simulink model "Longitudinal_new_modified"  (R2025b)
settings: Solver=VariableStepAuto  StartTime=0.0  StopTime=4  MaxStep=0.001  RelTol=1e-3
undefined symbols (not defined in the file): car, rad, s, Tau_1, Tau_2, Tau_3, Tau_4, Tau_EM, tyre
libraries: aerolibconvert2 x3, simulink x2
(part 2 of 2)

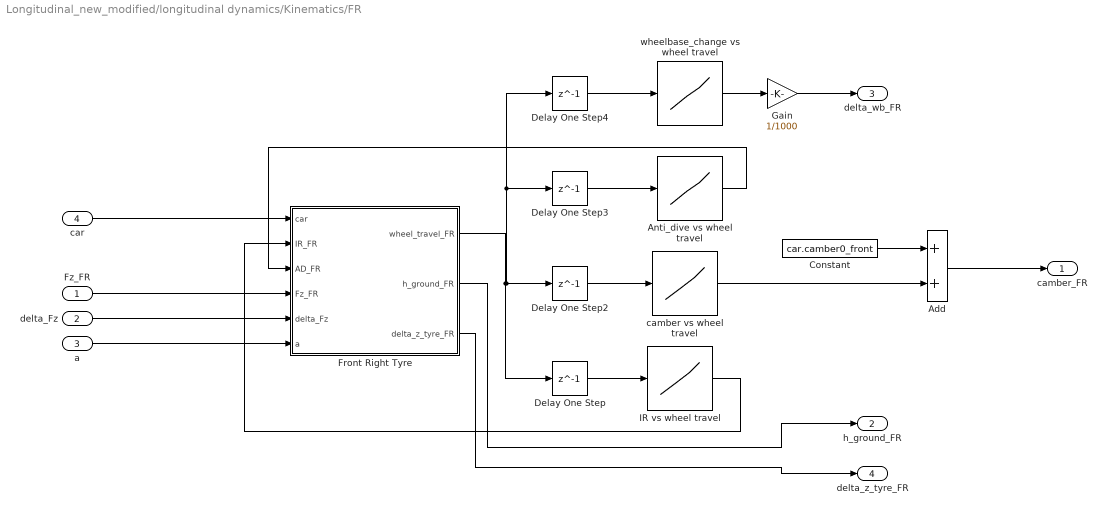
== system Longitudinal_new_modified/longitudinal dynamics/Kinematics/FR ==
  Fz_FR : Inport
  delta_Fz : Inport  Port=2
  a : Inport  Port=3
  car : Inport  Port=4
  Add : Sum
  Anti_dive vs wheel travel : Lookup_n-D  NumberOfTableDimensions=1  BreakpointsForDimension1=[-20;-19;-18;-17;-16;-15;-14;-13;-12;-11;-10;-9;-8;-7;-6;-5;-4;-3;-2;-1;0;1;2;3;4;5;6;7;8;9;10;11;12;13;14;15;16;17;18;19;20;21;22;23;24;25;26;27;28;29;30;31;32;33;34;35;36;37;38;39;40;41;42;43;44;45;46;47;48;49;50;51;52;53;54;55;56;57;58;59;60;61;62;63;64;65;66;67;68;69;70;71;72;73;74;75]  Table=[56.11;56.3;56.5;56.69;56.89;57.08;57.28;57.48;57.68;57.88;58.09;58.29;58.5;58.7;58.91;59.12;59.33;59.54;59.76;59.97;60.19;60.4;60.62;60.84;61.06;61.29;61.51;61.74;61.96;62.19;62.42;62.65;62.88;63.12;63.35;63.59;63.83;64.06999999999999;64.31;64.56;64.8;65.05;65.3;65.55;65.8;66.05;66.31;66.56999999999999;66.83;67.09;67.34999999999999;67.61;67.88;68.15000000000001;68.42;68.69;68.95999999999999;69.23999999999999;69.52;69.8;70.08;70.36;70.65000000000001;70.94;71.23;71.52;71.81;72.11;72.41;72.70999999999999;73.02;73.31999999999999;73.63;73.94;74.25;74.56999999999999;74.89;75.20999999999999;75.53;75.84999999999999;76.18000000000001;76.51000000000001;76.84999999999999;77.18000000000001;77.52;77.86;78.20999999999999;78.55;78.90000000000001;79.26000000000001;79.61;79.97;80.33;80.7;81.06;81.43000000000001]  InternalRulePriority=Speed  RndMeth=Simplest
  Constant : Constant  Value=car.camber0_front
  Delay One Step{,2..4} (4 alike) : Delay  DelayLength=1
  Front Right Tyre : MATLAB Function  TreatAsAtomicUnit=on
  Gain : Gain  Gain=1/1000
  IR vs wheel travel : Lookup_n-D  NumberOfTableDimensions=1  BreakpointsForDimension1=[-20;-19;-18;-17;-16;-15;-14;-13;-12;-11;-10;-9;-8;-7;-6;-5;-4;-3;-2;-1;0;1;2;3;4;5;6;7;8;9;10;11;12;13;14;15;16;17;18;19;20;21;22;23;24;25;26;27;28;29;30;31;32;33;34;35;36;37;38;39;40;41;42;43;44;45;46;47;48;49;50;51;52;53;54;55;56;57;58;59;60;61;62;63;64;65;66;67;68;69;70;71;72;73;74;75]  Table=[0.5620000000000001;0.562105263157895;0.562222222222222;0.5623529411764711;0.5625;0.562666666666667;0.5628571428571429;0.563076923076923;0.563333333333333;0.562727272727273;0.5629999999999999;0.563333333333333;0.5625;0.5628571428571429;0.563333333333333;0.5639999999999999;0.5625;0.563333333333333;0.5649999999999999;0.5600000000000001;0.5600000000000001;0.5600000000000001;0.5649999999999999;0.563333333333333;0.5625;0.5620000000000001;0.561666666666667;0.5614285714285711;0.56125;0.561111111111111;0.5610000000000001;0.560909090909091;0.560833333333333;0.560769230769231;0.5607142857142861;0.560666666666667;0.5600000000000001;0.5600000000000001;0.559444444444444;0.559473684210526;0.5590000000000001;0.559047619047619;0.558636363636364;0.558260869565217;0.5579166666666669;0.5576;0.5573076923076919;0.557037037037037;0.556785714285714;0.556551724137931;0.556333333333333;0.555806451612903;0.555625;0.555151515151515;0.554705882352941;0.554571428571429;0.554166666666667;0.553783783783784;0.553421052631579;0.553076923076923;0.55275;0.5524390243902439;0.551904761904762;0.551627906976744;0.551136363636364;0.550888888888889;0.550434782608696;0.55;0.549583333333333;0.549183673469388;0.5488;0.54843137254902;0.548076923076923;0.547547169811321;0.5472222222222221;0.546727272727273;0.546428571428571;0.545964912280702;0.54551724137931;0.545084745762712;0.544666666666667;0.544262295081967;0.543870967741935;0.543492063492063;0.543125;0.5426153846153851;0.542272727272727;0.5417910447761189;0.541323529411765;0.587971014492754;0.585285714285714;0.582676056338028;0.580277777777778;0.577808219178082;0.575405405405405;0.5732]  InternalRulePriority=Speed  RndMeth=Simplest
  camber vs wheel travel : Lookup_n-D  NumberOfTableDimensions=1  BreakpointsForDimension1=[-20;-19;-18;-17;-16;-15;-14;-13;-12;-11;-10;-9;-8;-7;-6;-5;-4;-3;-2;-1;0;1;2;3;4;5;6;7;8;9;10;11;12;13;14;15;16;17;18;19;20;21;22;23;24;25;26;27;28;29;30;31;32;33;34;35;36;37;38;39;40;41;42;43;44;45;46;47;48;49;50;51;52;53;54;55;56;57;58;59;60;61;62;63;64;65;66;67;68;69;70;71;72;73;74;75]  Table=[0.94910000000000005;0.90229999999999999;0.85550000000000004;0.80859999999999999;0.76160000000000005;0.71450000000000002;0.66739999999999999;0.62019999999999997;0.57299999999999995;0.52569999999999995;0.4783;0.43080000000000002;0.38319999999999999;0.33560000000000001;0.28789999999999999;0.24010000000000001;0.1923;0.14430000000000001;0.096299999999999997;0.0482;0;-0.048300000000000003;-0.096600000000000005;-0.14510000000000001;-0.19359999999999999;-0.2422;-0.29089999999999999;-0.3397;-0.3886;-0.43759999999999999;-0.48670000000000002;-0.53580000000000005;-0.58509999999999995;-0.63439999999999996;-0.68389999999999995;-0.73340000000000005;-0.78310000000000002;-0.83279999999999998;-0.88270000000000004;-0.93259999999999998;-0.98270000000000002;-1.0327999999999999;-1.0831;-1.1334;-1.1839;-1.2344999999999999;-1.2851999999999999;-1.3360000000000001;-1.3869;-1.4379;-1.4890000000000001;-1.5403;-1.5915999999999999;-1.6431;-1.6947000000000001;-1.7464;-1.7982;-1.8501000000000001;-1.9021999999999999;-1.9543999999999999;-2.0066999999999999;-2.0590999999999999;-2.1116999999999999;-2.1644000000000001;-2.2172000000000001;-2.2700999999999998;-2.3231999999999999;-2.3763999999999998;-2.4297;-2.4830999999999999;-2.5367000000000002;-2.5903999999999998;-2.6442999999999999;-2.6983000000000001;-2.7524000000000002;-2.8067000000000002;-2.8611;-2.9156;-2.9702999999999999;-3.0251000000000001;-3.0800999999999998;-3.1352000000000002;-3.1903999999999999;-3.2458;-3.3014000000000001;-3.3571;-3.4129;-3.4689000000000001;-3.5251000000000001;-3.5813999999999999;-3.6377999999999999;-3.6945000000000001;-3.7511999999999999;-3.8081;-3.8652000000000002;-3.9224999999999999]  InternalRulePriority=Speed  RndMeth=Simplest
  wheelbase_change vs wheel travel : Lookup_n-D  NumberOfTableDimensions=1  BreakpointsForDimension1=[-20;-19;-18;-17;-16;-15;-14;-13;-12;-11;-10;-9;-8;-7;-6;-5;-4;-3;-2;-1;0;1;2;3;4;5;6;7;8;9;10;11;12;13;14;15;16;17;18;19;20;21;22;23;24;25;26;27;28;29;30;31;32;33;34;35;36;37;38;39;40;41;42;43;44;45;46;47;48;49;50;51;52;53;54;55;56;57;58;59;60;61;62;63;64;65;66;67;68;69;70;71;72;73;74;75]  Table=[0.25;0.23999999999999999;0.22;0.20999999999999999;0.19;0.17999999999999999;0.16;0.14999999999999999;0.13;0.12;0.11;0.10000000000000001;0.080000000000000002;0.070000000000000007;0.059999999999999998;0.050000000000000003;0.040000000000000001;0.029999999999999999;0.02;0.01;0;-0.01;-0.02;-0.029999999999999999;-0.029999999999999999;-0.040000000000000001;-0.050000000000000003;-0.050000000000000003;-0.059999999999999998;-0.070000000000000007;-0.070000000000000007;-0.080000000000000002;-0.080000000000000002;-0.080000000000000002;-0.089999999999999997;-0.089999999999999997;-0.089999999999999997;-0.10000000000000001;-0.10000000000000001;-0.10000000000000001;-0.10000000000000001;-0.10000000000000001;-0.10000000000000001;-0.10000000000000001;-0.10000000000000001;-0.10000000000000001;-0.10000000000000001;-0.10000000000000001;-0.089999999999999997;-0.089999999999999997;-0.089999999999999997;-0.080000000000000002;-0.080000000000000002;-0.070000000000000007;-0.070000000000000007;-0.059999999999999998;-0.059999999999999998;-0.050000000000000003;-0.040000000000000001;-0.040000000000000001;-0.029999999999999999;-0.02;-0.01;0;0.01;0.02;0.029999999999999999;0.040000000000000001;0.050000000000000003;0.070000000000000007;0.080000000000000002;0.089999999999999997;0.11;0.12;0.13;0.14999999999999999;0.17000000000000001;0.17999999999999999;0.20000000000000001;0.22;0.23999999999999999;0.25;0.27000000000000002;0.28999999999999998;0.31;0.33000000000000002;0.34999999999999998;0.38;0.40000000000000002;0.41999999999999998;0.45000000000000001;0.46999999999999997;0.48999999999999999;0.52000000000000002;0.55000000000000004;0.56999999999999995]  InternalRulePriority=Speed  RndMeth=Simplest
  camber_FR : Outport
  h_ground_FR : Outport  Port=2
  delta_wb_FR : Outport  Port=3
  delta_z_tyre_FR : Outport  Port=4
  wires:
  Delay One Step2/1 -> camber vs wheel travel/1
  Front Right Tyre/1(wheel_travel_FR) -> Delay One Step/1, Delay One Step3/1, Delay One Step4/1, Delay One Step2/1
  Delay One Step/1 -> IR vs wheel travel/1
  IR vs wheel travel/1 -> Front Right Tyre/2(IR_FR)
  Front Right Tyre/2(h_ground_FR) -> h_ground_FR/1
  delta_Fz/1 -> Front Right Tyre/5(delta_Fz)
  Anti_dive vs wheel travel/1 -> Front Right Tyre/3(AD_FR)
  Delay One Step3/1 -> Anti_dive vs wheel travel/1
  Delay One Step4/1 -> wheelbase_change vs wheel travel/1
  wheelbase_change vs wheel travel/1 -> Gain/1
  Fz_FR/1 -> Front Right Tyre/4(Fz_FR)
  Front Right Tyre/3(delta_z_tyre_FR) -> delta_z_tyre_FR/1
  Constant/1 -> Add/1
  camber vs wheel travel/1 -> Add/2
  Add/1 -> camber_FR/1
  a/1 -> Front Right Tyre/6(a)
  car/1 -> Front Right Tyre/1(car)
  Gain/1 -> delta_wb_FR/1

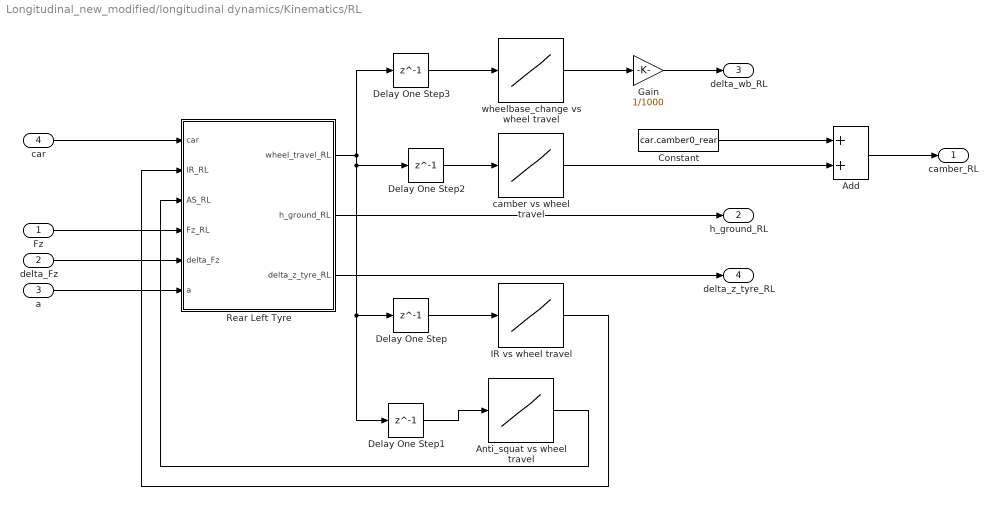
== system Longitudinal_new_modified/longitudinal dynamics/Kinematics/RL ==
  Fz : Inport
  delta_Fz : Inport  Port=2
  a : Inport  Port=3
  car : Inport  Port=4
  Add : Sum
  Anti_squat vs wheel travel : Lookup_n-D  NumberOfTableDimensions=1  BreakpointsForDimension1=[-20;-19;-18;-17;-16;-15;-14;-13;-12;-11;-10;-9;-8;-7;-6;-5;-4;-3;-2;-1;0;1;2;3;4;5;6;7;8;9;10;11;12;13;14;15;16;17;18;19;20;21;22;23;24;25;26;27;28;29;30;31;32;33;34;35;36;37;38;39;40;41;42;43;44;45;46;47;48;49;50;51;52;53;54;55;56;57;58;59;60;61;62;63;64;65;66;67;68;69;70;71;72;73;74;75]  Table=[54.63;54.63;54.63;54.63;54.63;54.64;54.64;54.64;54.65;54.65;54.66;54.66;54.67;54.67;54.68;54.69;54.69;54.7;54.71;54.71;54.72;54.73;54.74;54.75;54.75;54.76;54.77;54.78;54.79;54.8;54.81;54.82;54.83;54.84;54.85;54.87;54.88;54.89;54.9;54.91;54.92;54.94;54.95;54.96;54.97;54.99;55;55.01;55.03;55.04;55.05;55.07;55.08;55.1;55.11;55.12;55.14;55.15;55.17;55.18;55.2;55.21;55.22;55.24;55.25;55.27;55.28;55.3;55.31;55.33;55.34;55.36;55.37;55.38;55.4;55.41;55.43;55.44;55.46;55.47;55.48;55.5;55.51;55.52;55.54;55.55;55.56;55.58;55.59;55.6;55.61;55.62;55.64;55.65;55.66;55.67]  InternalRulePriority=Speed  RndMeth=Simplest
  Constant : Constant  Value=car.camber0_rear
  Delay One Step{,1..3} (4 alike) : Delay  DelayLength=1
  Gain : Gain  Gain=1/1000
  IR vs wheel travel : Lookup_n-D  NumberOfTableDimensions=1  BreakpointsForDimension1=[-20;-19;-18;-17;-16;-15;-14;-13;-12;-11;-10;-9;-8;-7;-6;-5;-4;-3;-2;-1;0;1;2;3;4;5;6;7;8;9;10;11;12;13;14;15;16;17;18;19;20;21;22;23;24;25;26;27;28;29;30;31;32;33;34;35;36;37;38;39;40;41;42;43;44;45;46;47;48;49;50;51;52;53;54;55;56;57;58;59;60;61;62;63;64;65;66;67;68;69;70;71;72;73;74;75]  Table=[0.78;0.78;0.78;0.78;0.78;0.78;0.78;0.78;0.78;0.78;0.78;0.78;0.78;0.78;0.78;0.78;0.78;0.78;0.78;0.78;0.78;0.78;0.78;0.78;0.78;0.78;0.78;0.78;0.78;0.78;0.78;0.78;0.78;0.78;0.78;0.78;0.78;0.78;0.78;0.78;0.78;0.78;0.78;0.78;0.78;0.78;0.78;0.78;0.78;0.78;0.78;0.78;0.78;0.78;0.78;0.78;0.78;0.78;0.78;0.78;0.78;0.78;0.78;0.78;0.78;0.78;0.78;0.78;0.78;0.78;0.78;0.78;0.78;0.78;0.78;0.78;0.78;0.78;0.78;0.78;0.78;0.78;0.78;0.78;0.78;0.78;0.78;0.78;0.78;0.78;0.78;0.78;0.78;0.78;0.78;0.78]  InternalRulePriority=Speed  RndMeth=Simplest
  Rear Left Tyre : MATLAB Function  TreatAsAtomicUnit=on
  camber vs wheel travel : Lookup_n-D  NumberOfTableDimensions=1  BreakpointsForDimension1=[-20;-19;-18;-17;-16;-15;-14;-13;-12;-11;-10;-9;-8;-7;-6;-5;-4;-3;-2;-1;0;1;2;3;4;5;6;7;8;9;10;11;12;13;14;15;16;17;18;19;20;21;22;23;24;25;26;27;28;29;30;31;32;33;34;35;36;37;38;39;40;41;42;43;44;45;46;47;48;49;50;51;52;53;54;55;56;57;58;59;60;61;62;63;64;65;66;67;68;69;70;71;72;73;74;75]  Table=[0.78749999999999998;0.74790000000000001;0.70840000000000003;0.66879999999999995;0.62929999999999997;0.58989999999999998;0.5504;0.51100000000000001;0.47160000000000002;0.43219999999999997;0.39279999999999998;0.35349999999999998;0.31419999999999998;0.27489999999999998;0.2356;0.1963;0.157;0.1177;0.0785;0.039199999999999999;0;-0.039199999999999999;-0.0785;-0.1177;-0.15690000000000001;-0.19620000000000001;-0.2354;-0.27460000000000001;-0.31390000000000001;-0.35310000000000002;-0.39240000000000003;-0.43159999999999998;-0.47089999999999999;-0.51019999999999999;-0.54949999999999999;-0.58879999999999999;-0.62809999999999999;-0.66739999999999999;-0.70679999999999998;-0.74619999999999997;-0.78559999999999997;-0.82499999999999996;-0.86450000000000005;-0.90390000000000004;-0.94340000000000002;-0.9829;-1.0225;-1.0621;-1.1016999999999999;-1.1414;-1.181;-1.2208000000000001;-1.2605;-1.3003;-1.3401000000000001;-1.3799999999999999;-1.4198999999999999;-1.4599;-1.4999;-1.54;-1.5801000000000001;-1.6202000000000001;-1.6604000000000001;-1.7007000000000001;-1.7410000000000001;-1.7814000000000001;-1.8218000000000001;-1.8623000000000001;-1.9028;-1.9434;-1.9841;-2.0247999999999999;-2.0655999999999999;-2.1065;-2.1474000000000002;-2.1884000000000001;-2.2294999999999998;-2.2706;-2.3117999999999999;-2.3531;-2.3944999999999999;-2.4359999999999999;-2.4775;-2.5190999999999999;-2.5608;-2.6025999999999998;-2.6444999999999999;-2.6863999999999999;-2.7284999999999999;-2.7706;-2.8128000000000002;-2.8552;-2.8976000000000002;-2.9401000000000002;-2.9826999999999999;-3.0255000000000001]  InternalRulePriority=Speed  RndMeth=Simplest
  wheelbase_change vs wheel travel : Lookup_n-D  NumberOfTableDimensions=1  BreakpointsForDimension1=[-20;-19;-18;-17;-16;-15;-14;-13;-12;-11;-10;-9;-8;-7;-6;-5;-4;-3;-2;-1;0;1;2;3;4;5;6;7;8;9;10;11;12;13;14;15;16;17;18;19;20;21;22;23;24;25;26;27;28;29;30;31;32;33;34;35;36;37;38;39;40;41;42;43;44;45;46;47;48;49;50;51;52;53;54;55;56;57;58;59;60;61;62;63;64;65;66;67;68;69;70;71;72;73;74;75]  Table=[-2.23;-2.1099999999999999;-2;-1.8899999999999999;-1.77;-1.6599999999999999;-1.55;-1.4299999999999999;-1.3200000000000001;-1.21;-1.1000000000000001;-0.98999999999999999;-0.88;-0.77000000000000002;-0.66000000000000003;-0.55000000000000004;-0.44;-0.33000000000000002;-0.22;-0.11;0;0.11;0.22;0.32000000000000001;0.42999999999999999;0.54000000000000004;0.64000000000000001;0.75;0.85999999999999999;0.95999999999999996;1.0700000000000001;1.1699999999999999;1.28;1.3799999999999999;1.49;1.5900000000000001;1.7;1.8;1.8999999999999999;2.0099999999999998;2.1099999999999999;2.21;2.3199999999999998;2.4199999999999999;2.52;2.6200000000000001;2.7200000000000002;2.8199999999999998;2.9199999999999999;3.02;3.1200000000000001;3.2200000000000002;3.3199999999999998;3.4199999999999999;3.52;3.6200000000000001;3.7200000000000002;3.8199999999999998;3.9199999999999999;4.0099999999999998;4.1100000000000003;4.21;4.3099999999999996;4.4000000000000004;4.5;4.5999999999999996;4.6900000000000004;4.79;4.8799999999999999;4.9800000000000004;5.0800000000000001;5.1699999999999999;5.2699999999999996;5.3600000000000003;5.4500000000000002;5.5499999999999998;5.6399999999999997;5.7400000000000002;5.8300000000000001;5.9199999999999999;6.0099999999999998;6.1100000000000003;6.2000000000000002;6.29;6.3799999999999999;6.4699999999999998;6.5700000000000003;6.6600000000000001;6.75;6.8399999999999999;6.9299999999999997;7.0199999999999996;7.1100000000000003;7.2000000000000002;7.29;7.3799999999999999]  InternalRulePriority=Speed  RndMeth=Simplest
  camber_RL : Outport
  h_ground_RL : Outport  Port=2
  delta_wb_RL : Outport  Port=3
  delta_z_tyre_RL : Outport  Port=4
  wires:
  Delay One Step2/1 -> camber vs wheel travel/1
  Rear Left Tyre/1(wheel_travel_RL) -> Delay One Step3/1, Delay One Step1/1, Delay One Step/1, Delay One Step2/1
  Delay One Step/1 -> IR vs wheel travel/1
  Anti_squat vs wheel travel/1 -> Rear Left Tyre/3(AS_RL)
  IR vs wheel travel/1 -> Rear Left Tyre/2(IR_RL)
  Delay One Step1/1 -> Anti_squat vs wheel travel/1
  delta_Fz/1 -> Rear Left Tyre/5(delta_Fz)
  Fz/1 -> Rear Left Tyre/4(Fz_RL)
  Delay One Step3/1 -> wheelbase_change vs wheel travel/1
  wheelbase_change vs wheel travel/1 -> Gain/1
  Rear Left Tyre/2(h_ground_RL) -> h_ground_RL/1
  Rear Left Tyre/3(delta_z_tyre_RL) -> delta_z_tyre_RL/1
  Add/1 -> camber_RL/1
  Constant/1 -> Add/1
  camber vs wheel travel/1 -> Add/2
  a/1 -> Rear Left Tyre/6(a)
  car/1 -> Rear Left Tyre/1(car)
  Gain/1 -> delta_wb_RL/1

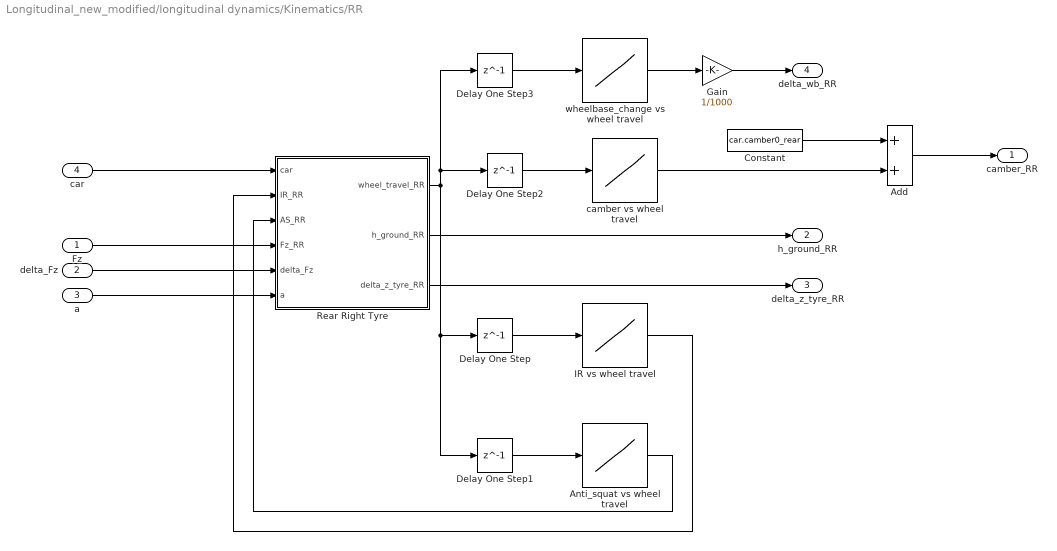
== system Longitudinal_new_modified/longitudinal dynamics/Kinematics/RR ==
  Fz : Inport
  delta_Fz : Inport  Port=2
  a : Inport  Port=3
  car : Inport  Port=4
  Add : Sum
  Anti_squat vs wheel travel : Lookup_n-D  NumberOfTableDimensions=1  BreakpointsForDimension1=[-20;-19;-18;-17;-16;-15;-14;-13;-12;-11;-10;-9;-8;-7;-6;-5;-4;-3;-2;-1;0;1;2;3;4;5;6;7;8;9;10;11;12;13;14;15;16;17;18;19;20;21;22;23;24;25;26;27;28;29;30;31;32;33;34;35;36;37;38;39;40;41;42;43;44;45;46;47;48;49;50;51;52;53;54;55;56;57;58;59;60;61;62;63;64;65;66;67;68;69;70;71;72;73;74;75]  Table=[54.63;54.63;54.63;54.63;54.63;54.64;54.64;54.64;54.65;54.65;54.66;54.66;54.67;54.67;54.68;54.69;54.69;54.7;54.71;54.71;54.72;54.73;54.74;54.75;54.75;54.76;54.77;54.78;54.79;54.8;54.81;54.82;54.83;54.84;54.85;54.87;54.88;54.89;54.9;54.91;54.92;54.94;54.95;54.96;54.97;54.99;55;55.01;55.03;55.04;55.05;55.07;55.08;55.1;55.11;55.12;55.14;55.15;55.17;55.18;55.2;55.21;55.22;55.24;55.25;55.27;55.28;55.3;55.31;55.33;55.34;55.36;55.37;55.38;55.4;55.41;55.43;55.44;55.46;55.47;55.48;55.5;55.51;55.52;55.54;55.55;55.56;55.58;55.59;55.6;55.61;55.62;55.64;55.65;55.66;55.67]  InternalRulePriority=Speed  RndMeth=Simplest
  Constant : Constant  Value=car.camber0_rear
  Delay One Step{,1..3} (4 alike) : Delay  DelayLength=1
  Gain : Gain  Gain=1/1000
  IR vs wheel travel : Lookup_n-D  NumberOfTableDimensions=1  BreakpointsForDimension1=[-20;-19;-18;-17;-16;-15;-14;-13;-12;-11;-10;-9;-8;-7;-6;-5;-4;-3;-2;-1;0;1;2;3;4;5;6;7;8;9;10;11;12;13;14;15;16;17;18;19;20;21;22;23;24;25;26;27;28;29;30;31;32;33;34;35;36;37;38;39;40;41;42;43;44;45;46;47;48;49;50;51;52;53;54;55;56;57;58;59;60;61;62;63;64;65;66;67;68;69;70;71;72;73;74;75]  Table=[0.78;0.78;0.78;0.78;0.78;0.78;0.78;0.78;0.78;0.78;0.78;0.78;0.78;0.78;0.78;0.78;0.78;0.78;0.78;0.78;0.78;0.78;0.78;0.78;0.78;0.78;0.78;0.78;0.78;0.78;0.78;0.78;0.78;0.78;0.78;0.78;0.78;0.78;0.78;0.78;0.78;0.78;0.78;0.78;0.78;0.78;0.78;0.78;0.78;0.78;0.78;0.78;0.78;0.78;0.78;0.78;0.78;0.78;0.78;0.78;0.78;0.78;0.78;0.78;0.78;0.78;0.78;0.78;0.78;0.78;0.78;0.78;0.78;0.78;0.78;0.78;0.78;0.78;0.78;0.78;0.78;0.78;0.78;0.78;0.78;0.78;0.78;0.78;0.78;0.78;0.78;0.78;0.78;0.78;0.78;0.78]  InternalRulePriority=Speed  RndMeth=Simplest
  Rear Right Tyre : MATLAB Function  TreatAsAtomicUnit=on
  camber vs wheel travel : Lookup_n-D  NumberOfTableDimensions=1  BreakpointsForDimension1=[-20;-19;-18;-17;-16;-15;-14;-13;-12;-11;-10;-9;-8;-7;-6;-5;-4;-3;-2;-1;0;1;2;3;4;5;6;7;8;9;10;11;12;13;14;15;16;17;18;19;20;21;22;23;24;25;26;27;28;29;30;31;32;33;34;35;36;37;38;39;40;41;42;43;44;45;46;47;48;49;50;51;52;53;54;55;56;57;58;59;60;61;62;63;64;65;66;67;68;69;70;71;72;73;74;75]  Table=[0.78749999999999998;0.74790000000000001;0.70840000000000003;0.66879999999999995;0.62929999999999997;0.58989999999999998;0.5504;0.51100000000000001;0.47160000000000002;0.43219999999999997;0.39279999999999998;0.35349999999999998;0.31419999999999998;0.27489999999999998;0.2356;0.1963;0.157;0.1177;0.0785;0.039199999999999999;0;-0.039199999999999999;-0.0785;-0.1177;-0.15690000000000001;-0.19620000000000001;-0.2354;-0.27460000000000001;-0.31390000000000001;-0.35310000000000002;-0.39240000000000003;-0.43159999999999998;-0.47089999999999999;-0.51019999999999999;-0.54949999999999999;-0.58879999999999999;-0.62809999999999999;-0.66739999999999999;-0.70679999999999998;-0.74619999999999997;-0.78559999999999997;-0.82499999999999996;-0.86450000000000005;-0.90390000000000004;-0.94340000000000002;-0.9829;-1.0225;-1.0621;-1.1016999999999999;-1.1414;-1.181;-1.2208000000000001;-1.2605;-1.3003;-1.3401000000000001;-1.3799999999999999;-1.4198999999999999;-1.4599;-1.4999;-1.54;-1.5801000000000001;-1.6202000000000001;-1.6604000000000001;-1.7007000000000001;-1.7410000000000001;-1.7814000000000001;-1.8218000000000001;-1.8623000000000001;-1.9028;-1.9434;-1.9841;-2.0247999999999999;-2.0655999999999999;-2.1065;-2.1474000000000002;-2.1884000000000001;-2.2294999999999998;-2.2706;-2.3117999999999999;-2.3531;-2.3944999999999999;-2.4359999999999999;-2.4775;-2.5190999999999999;-2.5608;-2.6025999999999998;-2.6444999999999999;-2.6863999999999999;-2.7284999999999999;-2.7706;-2.8128000000000002;-2.8552;-2.8976000000000002;-2.9401000000000002;-2.9826999999999999;-3.0255000000000001]  InternalRulePriority=Speed  RndMeth=Simplest
  wheelbase_change vs wheel travel : Lookup_n-D  NumberOfTableDimensions=1  BreakpointsForDimension1=[-20;-19;-18;-17;-16;-15;-14;-13;-12;-11;-10;-9;-8;-7;-6;-5;-4;-3;-2;-1;0;1;2;3;4;5;6;7;8;9;10;11;12;13;14;15;16;17;18;19;20;21;22;23;24;25;26;27;28;29;30;31;32;33;34;35;36;37;38;39;40;41;42;43;44;45;46;47;48;49;50;51;52;53;54;55;56;57;58;59;60;61;62;63;64;65;66;67;68;69;70;71;72;73;74;75]  Table=[-2.23;-2.1099999999999999;-2;-1.8899999999999999;-1.77;-1.6599999999999999;-1.55;-1.4299999999999999;-1.3200000000000001;-1.21;-1.1000000000000001;-0.98999999999999999;-0.88;-0.77000000000000002;-0.66000000000000003;-0.55000000000000004;-0.44;-0.33000000000000002;-0.22;-0.11;0;0.11;0.22;0.32000000000000001;0.42999999999999999;0.54000000000000004;0.64000000000000001;0.75;0.85999999999999999;0.95999999999999996;1.0700000000000001;1.1699999999999999;1.28;1.3799999999999999;1.49;1.5900000000000001;1.7;1.8;1.8999999999999999;2.0099999999999998;2.1099999999999999;2.21;2.3199999999999998;2.4199999999999999;2.52;2.6200000000000001;2.7200000000000002;2.8199999999999998;2.9199999999999999;3.02;3.1200000000000001;3.2200000000000002;3.3199999999999998;3.4199999999999999;3.52;3.6200000000000001;3.7200000000000002;3.8199999999999998;3.9199999999999999;4.0099999999999998;4.1100000000000003;4.21;4.3099999999999996;4.4000000000000004;4.5;4.5999999999999996;4.6900000000000004;4.79;4.8799999999999999;4.9800000000000004;5.0800000000000001;5.1699999999999999;5.2699999999999996;5.3600000000000003;5.4500000000000002;5.5499999999999998;5.6399999999999997;5.7400000000000002;5.8300000000000001;5.9199999999999999;6.0099999999999998;6.1100000000000003;6.2000000000000002;6.29;6.3799999999999999;6.4699999999999998;6.5700000000000003;6.6600000000000001;6.75;6.8399999999999999;6.9299999999999997;7.0199999999999996;7.1100000000000003;7.2000000000000002;7.29;7.3799999999999999]  InternalRulePriority=Speed  RndMeth=Simplest
  camber_RR : Outport
  h_ground_RR : Outport  Port=2
  delta_z_tyre_RR : Outport  Port=3
  delta_wb_RR : Outport  Port=4
  wires:
  Delay One Step2/1 -> camber vs wheel travel/1
  Rear Right Tyre/1(wheel_travel_RR) -> Delay One Step3/1, Delay One Step2/1, Delay One Step1/1, Delay One Step/1
  Delay One Step/1 -> IR vs wheel travel/1
  Anti_squat vs wheel travel/1 -> Rear Right Tyre/3(AS_RR)
  IR vs wheel travel/1 -> Rear Right Tyre/2(IR_RR)
  Delay One Step1/1 -> Anti_squat vs wheel travel/1
  Rear Right Tyre/2(h_ground_RR) -> h_ground_RR/1
  delta_Fz/1 -> Rear Right Tyre/5(delta_Fz)
  Rear Right Tyre/3(delta_z_tyre_RR) -> delta_z_tyre_RR/1
  Fz/1 -> Rear Right Tyre/4(Fz_RR)
  Delay One Step3/1 -> wheelbase_change vs wheel travel/1
  wheelbase_change vs wheel travel/1 -> Gain/1
  Constant/1 -> Add/1
  camber vs wheel travel/1 -> Add/2
  Add/1 -> camber_RR/1
  a/1 -> Rear Right Tyre/6(a)
  car/1 -> Rear Right Tyre/1(car)
  Gain/1 -> delta_wb_RR/1

== matlab function Longitudinal_new_modified/longitudinal dynamics/Min Fx solver/RR ==
  data: Fx_ICE input; Fx_RR output; Fx_tyre input; delta_Fx_RR output
function [Fx_RR, delta_Fx_RR] = fcn(Fx_ICE, Fx_tyre)

% add delta Fx for each tyre

if Fx_ICE<Fx_tyre
    Fx_RR = Fx_ICE;
    delta_Fx_RR = 0;
else 
    Fx_RR = Fx_tyre;
    delta_Fx_RR = Fx_ICE - Fx_tyre;
end

== matlab function Longitudinal_new_modified/longitudinal dynamics/Kinematics/FR/Front Right Tyre ==
  data: car input; wheel_travel_FR output; IR_FR input; AD_FR input; Fz_FR input; h_ground_FR output; delta_Fz input; delta_z_tyre_FR output; a input
function [wheel_travel_FR, h_ground_FR, delta_z_tyre_FR] = kinematics(car, IR_FR, AD_FR, Fz_FR, delta_Fz, a)

delta_z_tyre_FR = Fz_FR / car.k_tyre/1000; %m
% tyre vertical stiffness - kz_tyre - for front and rear tyres, look at buses
k_spring_ground_FR = (car.k_spring_front * IR_FR^2);

if a > 0 % under acceleration
    delta_z_spring_FR = Fz_FR / k_spring_ground_FR; % front axle
else % under braking
    delta_z_spring_FR = (Fz_FR - delta_Fz) / k_spring_ground_FR + delta_Fz * ((1-AD_FR/100)/k_spring_ground_FR) ; % front axle
end

%wheel center movement only due to spring deflection at ground. 
%to be used in the kineamtics block (camber, antidive, ir,...)
wheel_travel_FR = delta_z_spring_FR - car.z0_spring_front; % if negative it is bounce

%to be used to find the new height of the car from the ground
jounce_FR = delta_z_tyre_FR + delta_z_spring_FR - car.z0_front;
h_ground_FR = car.h0_ground_front - jounce_FR;

== matlab function Longitudinal_new_modified/Tyres/Front Left ==
  data: tyre_FL input; Fx output; Fy output
function [Fx, Fy] = fcn(tyre_FL)

y = u;

== matlab function Longitudinal_new_modified/longitudinal dynamics/Kinematics/RR/Rear Right Tyre ==
  data: car input; wheel_travel_RR output; IR_RR input; AS_RR input; Fz_RR input; h_ground_RR output; delta_Fz input; delta_z_tyre_RR output; a input
function [wheel_travel_RR, h_ground_RR, delta_z_tyre_RR]      = kinematics(car, IR_RR, AS_RR, Fz_RR, delta_Fz, a)

delta_z_tyre_RR = Fz_RR / car.k_tyre/1000; % tyre vertical stiffness - kz_tyre - for front and rear tyres, look at buses
k_spring_ground_RR = (car.k_spring_rear * IR_RR^2);

if a > 0 % under acceleration
    delta_z_spring_RR = (Fz_RR - delta_Fz) / k_spring_ground_RR + delta_Fz * ((1-AS_RR/100)/k_spring_ground_RR) ; % rear axle
else % under braking
    delta_z_spring_RR = Fz_RR / k_spring_ground_RR; % rear axle
end

%wheel center movement only due to spring deflection at ground. 
%to be used in the kineamtics block (camber, antidive, ir,...)
wheel_travel_RR = delta_z_spring_RR - car.z0_spring_rear; % if negative it is bounce

%to be used to find the new height of the car from the ground
jounce_RR = delta_z_tyre_RR + delta_z_spring_RR - car.z0_rear;
h_ground_RR = car.h0_ground_rear - jounce_RR;

== matlab function Longitudinal_new_modified/Tyres1/Front Right ==
  data: car input; SR input; Fx_FR output; Fz input; camber input
function Fx_FR = fcn(car,SR,Fz,camber)

% PAC2002 puro longitudinale (Fx vs k)
     Fz0 = car.tyre_Fz0;
     if Fz0 == 0, Fz0 = max(1, Fz); end
    dfz = (Fz - Fz0)/Fz0;

    pi0 = car.tyre_pi0;  % Pa nominale
    dpi = (car.tyre_pressure_front - pi0)/pi0;
    
Cx1 = car.tyre_Cx1;
Dx1 = car.tyre_Dx1;
Dx2 = car.tyre_Dx2;
Dx3 = car.tyre_Dx3;
Ex1 = car.tyre_Ex1;
Ex2 = car.tyre_Ex2;
Ex3 = car.tyre_Ex3;
Ex4 = car.tyre_Ex4;
Kx1 = car.tyre_Kx1;
Kx2 = car.tyre_Kx2;
Kx3 = car.tyre_Kx3;
Hx1 = car.tyre_Hx1;
Hx2 = car.tyre_Hx2;
Vx1 = car.tyre_Vx1;
Vx2 = car.tyre_Vx2;
px1 = car.tyre_px1;
px2 = car.tyre_px2;
px3 = car.tyre_px3;
px4 = car.tyre_px4;
lmux = car.tyre_lmux;


    gamma = camber*pi/180;
    mu = (Dx1 + Dx2*dfz) * (1 - Dx3*(gamma^2)) * (1 + px3*dpi + px4*dpi^2)*lmux;
    % mu = 1.4;

    D = mu * Fz;
    C = Cx1;
    K = Fz * (Kx1 + Kx2*dfz) * exp(Kx3*dfz) * (1 + px1*dpi + px2*dpi^2);
    B = K / (C*D + eps);

    SH = Hx1 + Hx2*dfz;
    SR  = SR + SH;

    E  = (Ex1 + Ex2*dfz + Ex3*dfz^2) * (1 - Ex4*sign(SR));
    SV = Fz * (Vx1 + Vx2*dfz);

    Fx0 = D * sin( C * atan( B*SR - E*(B*SR - atan(B*SR)) ) );
    Fx_FR = Fx0 + SV;

== matlab function Longitudinal_new_modified/longitudinal dynamics/Kinematics/FL/Front Left Tyre ==
  data: car input; wheel_travel_FL output; IR_FL input; AD_FL input; Fz_FL input; h_ground_FL output; delta_Fz input; delta_z_tyre_FL output; a input
function [wheel_travel_FL, h_ground_FL, delta_z_tyre_FL] = kinematics(car, IR_FL, AD_FL, Fz_FL, delta_Fz, a)

delta_z_tyre_FL = Fz_FL / car.k_tyre/1000; % tyre vertical stiffness - kz_tyre - for front and rear tyres, look at buses
k_spring_ground_FL = (car.k_spring_front * IR_FL^2);

if a > 0 % under acceleration
    delta_z_spring_FL = Fz_FL / k_spring_ground_FL; % front axle
else % under braking
    delta_z_spring_FL = (Fz_FL - delta_Fz) / k_spring_ground_FL + delta_Fz * ((1-AD_FL/100)/k_spring_ground_FL) ; % front axle
end

%wheel center movement only due to spring deflection at ground. 
%to be used in the kineamtics block (camber, antidive, ir,...)
wheel_travel_FL = delta_z_spring_FL - car.z0_spring_front; % if negative it is bounce

%to be used to find the new height of the car from the ground
jounce_FL = delta_z_tyre_FL + delta_z_spring_FL - car.z0_front;
h_ground_FL = car.h0_ground_front - jounce_FL;

== matlab function Longitudinal_new_modified/Tyres1/Rear Left ==
  data: car input; Fx_RL output; SR input; Fz input; camber input
function Fx_RL = fcn(car,SR,Fz,camber)

% PAC2002 puro longitudinale (Fx vs k)

     Fz0 = car.tyre_Fz0;
     if Fz0 == 0, Fz0 = max(1, Fz); end
    dfz = (Fz - Fz0)/Fz0;

    pi0 = car.tyre_pi0;  % Pa nominale
    dpi = (car.tyre_pressure_rear - pi0)/pi0;
    
Cx1 = car.tyre_Cx1;
Dx1 = car.tyre_Dx1;
Dx2 = car.tyre_Dx2;
Dx3 = car.tyre_Dx3;
Ex1 = car.tyre_Ex1;
Ex2 = car.tyre_Ex2;
Ex3 = car.tyre_Ex3;
Ex4 = car.tyre_Ex4;
Kx1 = car.tyre_Kx1;
Kx2 = car.tyre_Kx2;
Kx3 = car.tyre_Kx3;
Hx1 = car.tyre_Hx1;
Hx2 = car.tyre_Hx2;
Vx1 = car.tyre_Vx1;
Vx2 = car.tyre_Vx2;
px1 = car.tyre_px1;
px2 = car.tyre_px2;
px3 = car.tyre_px3;
px4 = car.tyre_px4;
lmux = car.tyre_lmux;


    gamma = camber*pi/180;
    mu = (Dx1 + Dx2*dfz) * (1 - Dx3*(gamma^2)) * (1 + px3*dpi + px4*dpi^2)*lmux;
    % mu = 1.4;

    D = mu * Fz;
    C = Cx1;
    K = Fz * (Kx1 + Kx2*dfz) * exp(Kx3*dfz) * (1 + px1*dpi + px2*dpi^2);
    B = K / (C*D + eps);

    SH = Hx1 + Hx2*dfz;
    SR  = SR + SH;

    E  = (Ex1 + Ex2*dfz + Ex3*dfz^2) * (1 - Ex4*sign(SR));
    SV = Fz * (Vx1 + Vx2*dfz);

    Fx0 = D * sin( C * atan( B*SR - E*(B*SR - atan(B*SR)) ) );
    Fx_RL = Fx0 + SV;

== matlab function Longitudinal_new_modified/Tyres1/Rear Right ==
  data: car input; Fx_RR output; SR input; Fz input; camber input
function Fx_RR = fcn(car,SR,Fz,camber)

% PAC2002 puro longitudinale (Fx vs k)

     Fz0 = car.tyre_Fz0;
     if Fz0 == 0, Fz0 = max(1, Fz); end
    dfz = (Fz - Fz0)/Fz0;

    pi0 = car.tyre_pi0;  % Pa nominale
    dpi = (car.tyre_pressure_rear - pi0)/pi0;
    
Cx1 = car.tyre_Cx1;
Dx1 = car.tyre_Dx1;
Dx2 = car.tyre_Dx2;
Dx3 = car.tyre_Dx3;
Ex1 = car.tyre_Ex1;
Ex2 = car.tyre_Ex2;
Ex3 = car.tyre_Ex3;
Ex4 = car.tyre_Ex4;
Kx1 = car.tyre_Kx1;
Kx2 = car.tyre_Kx2;
Kx3 = car.tyre_Kx3;
Hx1 = car.tyre_Hx1;
Hx2 = car.tyre_Hx2;
Vx1 = car.tyre_Vx1;
Vx2 = car.tyre_Vx2;
px1 = car.tyre_px1;
px2 = car.tyre_px2;
px3 = car.tyre_px3;
px4 = car.tyre_px4;
lmux = car.tyre_lmux;


    gamma = camber*pi/180;
    mu = (Dx1 + Dx2*dfz) * (1 - Dx3*(gamma^2)) * (1 + px3*dpi + px4*dpi^2)*lmux;
    % mu = 1.4;

    D = mu * Fz;
    C = Cx1;
    K = Fz * (Kx1 + Kx2*dfz) * exp(Kx3*dfz) * (1 + px1*dpi + px2*dpi^2);
    B = K / (C*D + eps);

    SH = Hx1 + Hx2*dfz;
    SR  = SR + SH;

    E  = (Ex1 + Ex2*dfz + Ex3*dfz^2) * (1 - Ex4*sign(SR));
    SV = Fz * (Vx1 + Vx2*dfz);

    Fx0 = D * sin( C * atan( B*SR - E*(B*SR - atan(B*SR)) ) );
    Fx_RR = Fx0 + SV;

== matlab function Longitudinal_new_modified/Powertrain/Clutch/MATLAB Function ==
  data: threshold input; w_out output; w_rear_in input; w_rear_out output
function [w_out, w_rear_out] = fcn(threshold, w_rear_in)

persistent isZero   % flag that stays true once threshold is reached

% Initialize the flag the first time the function is called
if isempty(isZero)
    isZero = false;
end

if w_rear_in >= threshold
    isZero = true;
end

% Output logic
if isZero
    w_out = 0;
    w_rear_out = w_rear_in;
else
    w_out = threshold;
    w_rear_out = 0;
end

end

== matlab function Longitudinal_new_modified/longitudinal dynamics/Fx powertrain calculation/RR ==
  data: delta input; Fz input; Fx_ICE_RR output; T input; J_r input; a input; R input
function Fx_ICE_RR = fcn(delta, Fz, T, J_r, a, R)

Fx_ICE_RR = (T - Fz * delta - J_r * a / R) / R ; % J - parameter for each tyre - J_f & J_r

== matlab function Longitudinal_new_modified/longitudinal dynamics/Fx powertrain calculation/FR ==
  data: Fz input; delta input; Fx_EM_FR output; T input; J_f input; a input; R input
function Fx_EM_FR = fcn(Fz, delta, T, J_f, a, R)

Fx_EM_FR = (T - Fz * delta - J_f * a / R) / R ; % J - parameter for each tyre - J_f & J_r

== matlab function Longitudinal_new_modified/longitudinal dynamics/Fx powertrain calculation/RL ==
  data: Fz input; T input; Fx_ICE_RL output; delta input; a input; J_r input; R input
function Fx_ICE_RL = fcn(Fz, T, delta, a, J_r, R)

Fx_ICE_RL = (T - Fz * delta - J_r * a / R) / R ; % J - parameter for each tyre - J_f & J_r

== matlab function Longitudinal_new_modified/longitudinal dynamics/Min Fx solver/RL ==
  data: Fx_ICE input; Fx_RL output; Fx_tyre input; delta_Fx_RL output
function [Fx_RL, delta_Fx_RL] = fcn(Fx_ICE, Fx_tyre)

% add delta Fx for each tyre

if Fx_ICE<Fx_tyre
    Fx_RL = Fx_ICE;
    delta_Fx_RL = 0;
else 
    Fx_RL = Fx_tyre;
    delta_Fx_RL = Fx_ICE - Fx_tyre;
end

== matlab function Longitudinal_new_modified/longitudinal dynamics/Min Fx solver/FR ==
  data: Fx_EM input; Fx_FR output; Fx_tyre input; delta_Fx_FR output
function [Fx_FR, delta_Fx_FR] = fcn(Fx_EM, Fx_tyre)

% add delta Fx for each tyre

if Fx_EM<Fx_tyre
    Fx_FR = Fx_EM;
    delta_Fx_FR = 0;
else 
    Fx_FR = Fx_tyre;
    delta_Fx_FR = Fx_EM - Fx_tyre;
end

== matlab function Longitudinal_new_modified/longitudinal dynamics/Min Fx solver/FL ==
  data: Fx_EM input; Fx_FL output; Fx_tyre input; delta_Fx_FL output
function [Fx_FL, delta_Fx_FL] = fcn(Fx_EM, Fx_tyre)

% add delta Fx for each tyre

if Fx_EM<Fx_tyre
    Fx_FL = Fx_EM;
    delta_Fx_FL = 0;
else 
    Fx_FL = Fx_tyre;
    delta_Fx_FL = Fx_EM - Fx_tyre;
end

== matlab function Longitudinal_new_modified/Powertrain/Driver model - gear selection/MATLAB Function3 ==
  settings: updateMethod=DISCRETE
  data: gear_trigger output; car input; gear_out output; v input
function [gear_trigger, gear_out] = change_gear(car, v)
%#codegen
% Selettore marcia per test di accelerazione
% - Si parte SEMPRE in 2a
% - Trigger di cambiata = impulso di un passo

    % --- stato interno: marcia attuale ---
    persistent gear
    if isempty(gear)
        gear = 2;                   % partenza in seconda
    end

    % parametri (R non ti serve qui ma lo lascio per completezza)
    R = car.R;
    v_thresh_up = [0, 24.9444, 1000];
    v_thresh_down = [0, 18, 30]; 
    tau      = [13.8304, 9.9320, 8.5118, 7.4490];
    nGearMax = numel(tau);

    % default: niente cambiata
    gear_trigger = 0;
    gear_out     = gear;

    % se sono già in ultima marcia non faccio nulla
    if gear >= nGearMax
        return;
    end

    % logica upshift: quando supero la soglia della marcia attuale
    if v >= v_thresh_up(gear)
        gear = gear + 1;
        gear_trigger = 1;           % impulso di cambiata
    end

    % logica downshift
    if gear > 1 && v <= v_down(gear)
        gear = gear - 1;
        gear_trigger = -1;
    end

    gear_out = gear;
end

== matlab function Longitudinal_new_modified/Tyres1/Front Left ==
  data: car input; Fx_FL output; SR input; Fz input; camber input
function Fx_FL = fcn(car,SR,Fz,camber)

% PAC2002 puro longitudinale (Fx vs k)

     Fz0 = car.tyre_Fz0;
     if Fz0 == 0, Fz0 = max(1, Fz); end
    dfz = (Fz - Fz0)/Fz0;

    pi0 = car.tyre_pi0;  % Pa nominale
    dpi = (car.tyre_pressure_front - pi0)/pi0;
    
Cx1 = car.tyre_Cx1;
Dx1 = car.tyre_Dx1;
Dx2 = car.tyre_Dx2;
Dx3 = car.tyre_Dx3;
Ex1 = car.tyre_Ex1;
Ex2 = car.tyre_Ex2;
Ex3 = car.tyre_Ex3;
Ex4 = car.tyre_Ex4;
Kx1 = car.tyre_Kx1;
Kx2 = car.tyre_Kx2;
Kx3 = car.tyre_Kx3;
Hx1 = car.tyre_Hx1;
Hx2 = car.tyre_Hx2;
Vx1 = car.tyre_Vx1;
Vx2 = car.tyre_Vx2;
px1 = car.tyre_px1;
px2 = car.tyre_px2;
px3 = car.tyre_px3;
px4 = car.tyre_px4;
lmux = car.tyre_lmux;


    gamma = camber*pi/180;
    mu = (Dx1 + Dx2*dfz) * (1 - Dx3*(gamma^2)) * (1 + px3*dpi + px4*dpi^2)*lmux;
    % mu = 1.4;

    D = mu * Fz;
    C = Cx1;
    K = Fz * (Kx1 + Kx2*dfz) * exp(Kx3*dfz) * (1 + px1*dpi + px2*dpi^2);
    B = K / (C*D + eps);

    SH = Hx1 + Hx2*dfz;
    SR  = SR + SH;

    E  = (Ex1 + Ex2*dfz + Ex3*dfz^2) * (1 - Ex4*sign(SR));
    SV = Fz * (Vx1 + Vx2*dfz);

    Fx0 = D * sin( C * atan( B*SR - E*(B*SR - atan(B*SR)) ) );
    Fx_FL = Fx0 + SV;

== matlab function Longitudinal_new_modified/longitudinal dynamics/Fx equilibrium ==
  data: Drag output; Fz_FL output; a input; Fz_RR output; Fz_RL output; Fz_FR output; delta_Fz output; v input; Cx input; Cz input; delta_wb_front input; delta_wb_rear input; car input
function [Drag, Fz_FL, Fz_RR, Fz_RL, Fz_FR, delta_Fz] = fx_equilibrium(a, v, Cx, Cz, delta_wb_front, delta_wb_rear,car)

wb = car.wb0 + delta_wb_front + delta_wb_rear; %m

Downforce = 0.5 * car.rho * Cz * car.frontal_area * v ^ 2; % downforce N
Drag = 0.5 * car.rho * Cx * car.frontal_area * v ^ 2; % drag N
M_aero = Drag * (car.h_cp - car.h_cog) - Downforce * (car.lf - car.x_cp); %Nm

delta_Fz = car.m * a * car.h_cog / wb + Drag * car.h_cog / wb - M_aero / wb; %N
delta_Fz=delta_Fz/2;
%J_f è di una singola ruota
%J_r totale da ruota a motore ICE
Fz_front = -(car.m * a + Drag) * car.h_cog / wb + (car.m * car.g + Downforce) * (car.lr + delta_wb_rear - car.delta) / wb - M_aero / wb - car.J_f*2* a / (car.R * wb); %N  (verificare J_f*4 oppure J_f*2!!!!!!!!!!!)

if Fz_front <= 0
    Fz_front = 0;
end

Fz_FR = Fz_front / 2 ;
Fz_FL = Fz_FR ;

Fz_rear = (car.m * a + Drag) * car.h_cog / wb + (car.m * car.g + Downforce) * (car.lf + delta_wb_front + car.delta) / wb + M_aero / wb + car.J_r * a / (car.R * wb); %N

if Fz_rear <= 0
    Fz_rear = 0;
end

Fz_RL = Fz_rear / 2;
Fz_RR = Fz_RL ;

== matlab function Longitudinal_new_modified/longitudinal dynamics/Fx powertrain calculation/FL ==
  data: delta input; R input; Fz input; J_f input; Fx_EM_FL output; T input; a input
function Fx_EM_FL = fcn(delta, R, Fz, J_f, T, a)

Fx_EM_FL = (T - Fz * delta - J_f * a / R) / R ; %N
% J - parameter for each tyre - J_f & J_r

== matlab function Longitudinal_new_modified/Tyres/Rear Right ==
  data: tyre_RR input; Fx output; Fy output
function [Fx, Fy] = fcn(tyre_RR)

y = u;

== matlab function Longitudinal_new_modified/Tyres/Front Right ==
  data: SR input; tyre input; Fx output; p input; Fz input; camber input
function Fx = fcn(SR,tyre,p,Fz,camber)

% PAC2002 puro longitudinale (Fx vs k)

     Fz0 = tyre.Fz0;
     if Fz0 == 0, Fz0 = max(1, Fz); end
    dfz = (Fz - Fz0)/Fz0;

    pi0 = tyre.pi0;  % Pa nominale
    dpi = (p - pi0)/pi0;
    
    Cx1 = tyre.Cx1;
    Dx1 = tyre.Dx1;
    Dx2 = tyre.Dx2;
    Dx3 = tyre.Dx3;
    Ex1 = tyre.Ex1;
    Ex2 = tyre.Ex2;
    Ex3 = tyre.Ex3;
    Ex4 = tyre.Ex4;
    Kx1 = tyre.Kx1;
    Kx2 = tyre.Kx2;
    Kx3 = tyre.Kx3;
    Hx1 = tyre.Hx1;
    Hx2 = tyre.Hx2;
    Vx1 = tyre.Vx1;
    Vx2 = tyre.Vx2;
    px1 = tyre.px1;
    px2 = tyre.px2;
    px3 = tyre.px3;
    px4 = tyre.px4;
    lmux = tyre.lmux;

    gamma = camber*pi/180;
    mu = (Dx1 + Dx2*dfz) * (1 - Dx3*(gamma^2)) * (1 + px3*dpi + px4*dpi^2)*lmux;
    % mu = 1.4;

    D = mu * Fz;
    C = Cx1;
    K = Fz * (Kx1 + Kx2*dfz) * exp(Kx3*dfz) * (1 + px1*dpi + px2*dpi^2);
    B = K / (C*D + eps);

    SH = Hx1 + Hx2*dfz;
    SR  = SR + SH;

    E  = (Ex1 + Ex2*dfz + Ex3*dfz^2) * (1 - Ex4*sign(SR));
    SV = Fz * (Vx1 + Vx2*dfz);

    Fx0 = D * sin( C * atan( B*SR - E*(B*SR - atan(B*SR)) ) );
    Fx = Fx0 + SV;

== matlab function Longitudinal_new_modified/Tyres/Rear Left ==
  data: tyre_RL input; Fx output; Fy output
function [Fx, Fy] = fcn(tyre_RL)

y = u;

== matlab function Longitudinal_new_modified/longitudinal dynamics/Kinematics/RL/Rear Left Tyre ==
  data: car input; wheel_travel_RL output; IR_RL input; AS_RL input; Fz_RL input; h_ground_RL output; delta_Fz input; delta_z_tyre_RL output; a input
function [wheel_travel_RL, h_ground_RL, delta_z_tyre_RL]      = kinematics(car, IR_RL, AS_RL, Fz_RL, delta_Fz, a)

delta_z_tyre_RL = Fz_RL / car.k_tyre/1000; % tyre vertical stiffness - kz_tyre - for front and rear tyres, look at buses
k_spring_ground_RL = (car.k_spring_rear * IR_RL^2);

if a > 0 % under acceleration
    delta_z_spring_RL = (Fz_RL - delta_Fz) / k_spring_ground_RL + delta_Fz * ((1-AS_RL/100)/k_spring_ground_RL) ; % rear axle
else % under braking
    delta_z_spring_RL = Fz_RL / k_spring_ground_RL; % rear axle
end

%wheel center movement only due to spring deflection at ground. 
%to be used in the kineamtics block (camber, antidive, ir,...)
wheel_travel_RL = delta_z_spring_RL - car.z0_spring_rear; % if negative it is bounce

%to be used to find the new height of the car from the ground
jounce_RL = delta_z_tyre_RL + delta_z_spring_RL - car.z0_rear;
h_ground_RL = car.h0_ground_rear - jounce_RL;
